simulink model "PIDa"  (Simulink 7.9)
settings: Solver=ode45  StartTime=0.0  StopTime=10  RelTol=1e-3
settings Model: Creator=Vaio  LastModifiedBy=Vaio

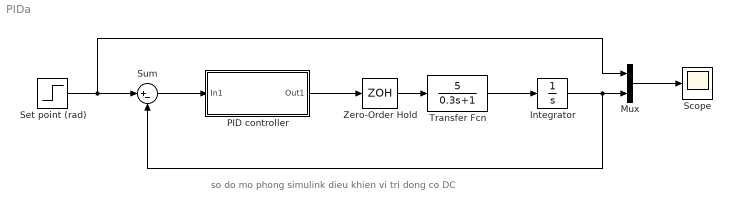
== system PIDa ==
  note: so do mo phong simulink dieu khien vi tri dong co DC
  Integrator : Integrator
  Mux : Mux  Inputs=2
  PID controller : Subsystem
  Scope : Scope
  Set point (rad) : Step  Time=0  After=100  SampleTime=0.005
  Sum : Sum  Inputs=|+-
  Transfer Fcn : TransferFcn  Numerator=[5]  Denominator=[0.3 1]
  Zero-Order Hold : ZeroOrderHold  SampleTime=0.005
  wires:
  Set point (rad)/1 -> Mux/1, Sum/1
  Zero-Order Hold/1 -> Transfer Fcn/1
  Transfer Fcn/1 -> Integrator/1
  Integrator/1 -> Mux/2, Sum/2
  Mux/1 -> Scope/1
  Sum/1 -> PID controller/1(In1)
  PID controller/1(Out1) -> Zero-Order Hold/1

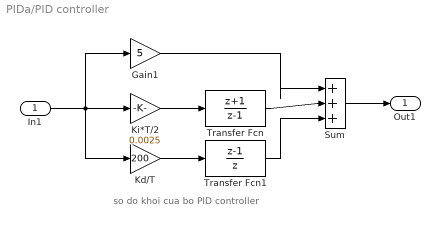
== system PIDa/PID controller ==
  note: so do khoi cua bo PID controller
  In1 : Inport
  Gain1 : Gain  Gain=5  SampleTime=0.005
  Kd/T : Gain  Gain=200  SampleTime=0.005
  Ki*T/2 : Gain  Gain=0.0025  SampleTime=0.005
  Sum : Sum  Inputs=|+++
  Transfer Fcn : DiscreteTransferFcn  Numerator=[1 1]  Denominator=[1 -1]  SampleTime=0.005
  Transfer Fcn1 : DiscreteTransferFcn  Numerator=[1 -1]  Denominator=[1 0]  SampleTime=0.005
  Out1 : Outport
  wires:
  In1/1 -> Gain1/1, Ki*T/2/1, Kd/T/1
  Ki*T/2/1 -> Transfer Fcn/1
  Kd/T/1 -> Transfer Fcn1/1
  Transfer Fcn/1 -> Sum/2
  Sum/1 -> Out1/1
  Transfer Fcn1/1 -> Sum/3
  Gain1/1 -> Sum/1
